simulink model "TA2445"  (R2022a)
settings: Solver=VariableStepAuto  StartTime=0.0  StopTime=51.5  MaxStep=0.01  RelTol=1e-3
model workspace (MAT data in the model file):
  IPTGconc = 0.0436365842371
  KE = 0.00336436543315
  XG0 = 0.005
  XG_max = 5.67988463796
  aE = 0.0190178810874
  dA = 0.148862069804
  k1 = 0.452621114798
  k2 = 1
  k3 = 2
  kA = 1913.69174642
  n0 = 4.80868240092
  rleak = 0.0606632472304
settings Model: Creator=tomok  LastModifiedBy=tomok

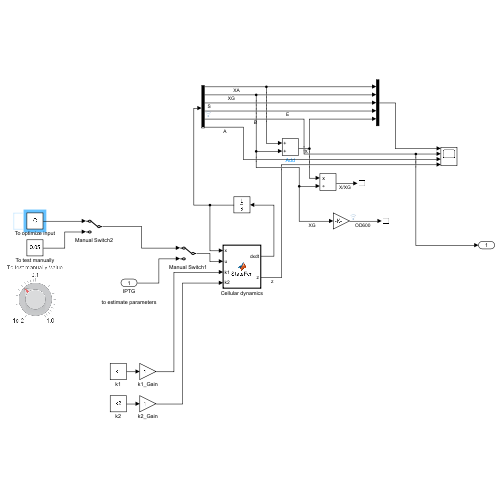
[thumbnail: Simulink's stored preview of the top-level diagram]
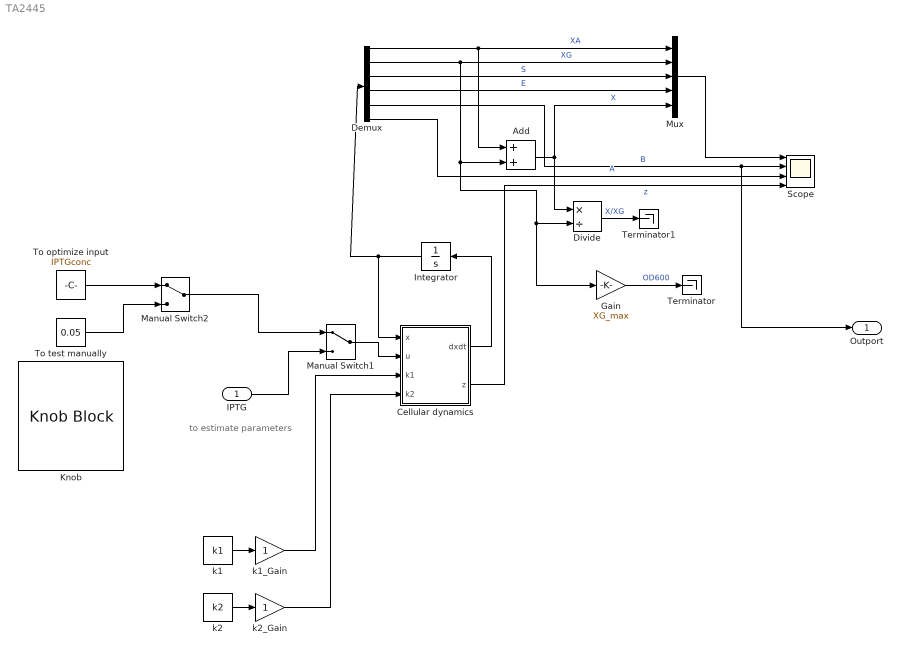
== system TA2445 ==
  note: to estimate parameters
  IPTG : Inport
  Add : Sum
  Cellular dynamics : MATLAB Function  TreatAsAtomicUnit=on
  Demux : Demux  Outputs=6
  Divide : Product  Inputs=*/
  Gain : Gain  Gain=XG_max
  Integrator : Integrator  InitialCondition=[n0*XG0; XG0; 1-n0*XG0-XG0; 0; 0; 0.01]
  Knob : KnobBlock  ScaleMin=0.01  ScaleMax=1  ScaleType=Log
  Manual Switch1 : ManualSwitch
  Manual Switch2 : ManualSwitch
  Mux : Mux  Inputs=5
  Scope : Scope  NumInputPorts=4
  Terminator : Terminator
  Terminator1 : Terminator
  To optimize input : Constant  Value=IPTGconc
  To test manually : Constant  Value=0.05
  k1 : Constant  Value=k1
  k1_Gain : Gain
  k2 : Constant  Value=k2
  k2_Gain : Gain
  Outport : Outport
  wires:
  Cellular dynamics/1(dxdt) -> Integrator/1
  Integrator/1 -> Demux/1, Cellular dynamics/1(x)
  Demux/1 -> Add/1, Mux/1  "XA"
  Demux/2 -> Add/2, Gain/1, Divide/2, Mux/2  "XG"
  Demux/3 -> Mux/3  "S"
  Add/1 -> Divide/1, Mux/5  "X"
  Divide/1 -> Terminator1/1  "X/XG"
  Mux/1 -> Scope/1
  To test manually/1 -> Manual Switch2/2
  Demux/4 -> Mux/4  "E"
  Demux/5 -> Outport/1, Scope/2  "B"
  IPTG/1 -> Manual Switch1/2
  Manual Switch1/1 -> Cellular dynamics/2(u)
  Gain/1 -> Terminator/1  "OD600"
  Cellular dynamics/2(z) -> Scope/4  "z"
  To optimize input/1 -> Manual Switch2/1
  Manual Switch2/1 -> Manual Switch1/1
  k2_Gain/1 -> Cellular dynamics/4(k2)
  k2/1 -> k2_Gain/1
  k1_Gain/1 -> Cellular dynamics/3(k1)
  k1/1 -> k1_Gain/1
  Demux/6 -> Scope/3  "A"

== matlab function TA2445/Cellular dynamics ==
  data: x input; dxdt output; u input; k3 parameter; rleak parameter; aE parameter; KE parameter; z output; kA parameter; dA parameter; k1 input; k2 input
function [dxdt,z] = StateFcn(x,u,k3, rleak, aE, KE, kA, dA, k1, k2)
%% Parameters
% k1 = 0.5;
% k2 = 1;
% k3 = 2;
% rleak = 0.3;
% aE = 0.3;
% KE = 0.2;

% kA = 10000;
% dA = 0.4;

% fixed parameters of the promoter response
KA = 1.596;
Ku = 0.02268;
nA = 1.752;
nu = 1.597;

%% Input variables and feed concentration

%% State variables
XA = x(1);
XG = x(2);
S = x(3);
E = x(4);
% B = x(5);
A = x(6);

%% Promoter response
z = (A^nA/(A^nA + KA^nA))*(u^nu/(u^nu + Ku^nu));

%% reaction rates
v1 = k1*S*(XA + XG + E)*(1 - (1 - rleak)*z); % substrate uptake
v2 = k2*XA*(XG + E);       % biomass formation (growth)
v3 = k3*(E/(E + KE))*XG;

%% ODEs
dXAdt = v1 - v2;
dXGdt = v2*(1 - aE*z);
dSdt = -v1;
dEdt = v2*aE*z;
dBdt = v3;
dAdt = kA*XG*z - dA*A;

dxdt = [dXAdt; dXGdt; dSdt; dEdt; dBdt; dAdt];

% lower limit of states
dxdt(x < 0 & dxdt < 0) = 0;
end
